simulink model "guitarraDistorcion"  (R2014a)
settings: Solver=ode45  StartTime=0.0  StopTime=inf  RelTol=1e-3
undefined symbols (not defined in the file): dfilt
libraries: dsparch4 x1, dspsrcs4 x1, dspsnks4 x1
settings Model: Creator=gbtom  LastModifiedBy=gbtom

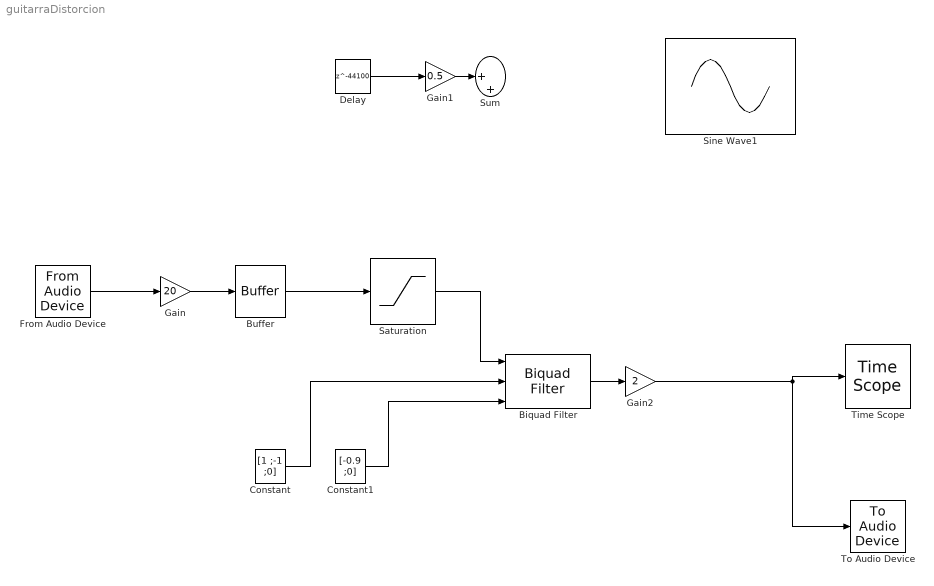
== system guitarraDistorcion ==
  Biquad Filter : dsparch4/Biquad Filter  IIRFiltStruct=Direct form II transposed  CoeffSource=Specify via dialog  BiQuadCoeffs=[1 0.3 0.4 1 0.1 0.2]  a0Flag=Warning  IC=0  ICnum=0  ICden=0  InputProcessing=Columns as channels (frame based)  denAccumFracLength=30  denProdOutputFracLength=30  secondMemoryFracLength=15  roundingMode=Floor  overflowMode=off  ScaleValues=1  optimizeScaleValues=on  ScaleValueMode=Assume all are unity and optimize  scaleValueFracLength=14  FilterSource=Input port(s)  dfiltObjectName=dfilt.df2tsos([1 0.3 0.4],[1 0.1 0.2])
  Buffer : Buffer  N=1024  TreatMby1Signals=One channel
  Constant : Constant  Value=[1 ;-1 ;0]  VectorParams1D=off
  Constant1 : Constant  Value=[-0.9 ;0]  VectorParams1D=off
  Delay : Delay  DelayLength=44100  InitialCondition=0  InputProcessing=Columns as channels (frame based)
  From Audio Device : dspsrcs4/From Audio Device  deviceName=Línea de entrada (3- BEHRINGER USB WDM AUDIO 2.8.40)  numChannels=1  sampleRate=44100  deviceDatatype=Determine from output data type  autoBufferSize=on  bufferSize=4096  queueDuration=1.0  frameSize=1024  outputDatatype=double  defaultInputChannelMapping=on  inputChannelMapping=1:2
  Gain : Gain  Gain=20
  Gain1 : Gain  Gain=0.5
  Gain2 : Gain  Gain=2
  Saturation : Saturate  UpperLimit=0.1  LowerLimit=-0.2
  Sine Wave1 : Sin  SineType=Sample based  Samples=150  SampleTime=1/44100
  Sum : Sum  Inputs=|++
  Time Scope : TimeScope  DefaultConfigurationName=spbscopes.TimeScopeBlockCfg
  To Audio Device : dspsnks4/To Audio Device  deviceName=Default  inheritSampleRate=off  sampleRate=44100  deviceDatatype=Determine from input data type  autoBufferSize=on  bufferSize=4096  queueDuration=1.0  defaultOutputChannelMapping=on  outputChannelMapping=1:2
  wires:
  From Audio Device/1 -> Gain/1
  Buffer/1 -> Saturation/1
  Delay/1 -> Gain1/1
  Gain1/1 -> Sum/1
  Constant/1 -> Biquad Filter/2
  Constant1/1 -> Biquad Filter/3
  Biquad Filter/1 -> Gain2/1
  Saturation/1 -> Biquad Filter/1
  Gain2/1 -> To Audio Device/1, Time Scope/1
  Gain/1 -> Buffer/1
